simulink subsystem "IMU"  (R2025b)
settings: Solver=VariableStepAuto  StartTime=0.0  StopTime=10.0  RelTol=1e-3
libraries: simulink x1
settings Model: Creator=diego  LastModifiedBy=diego

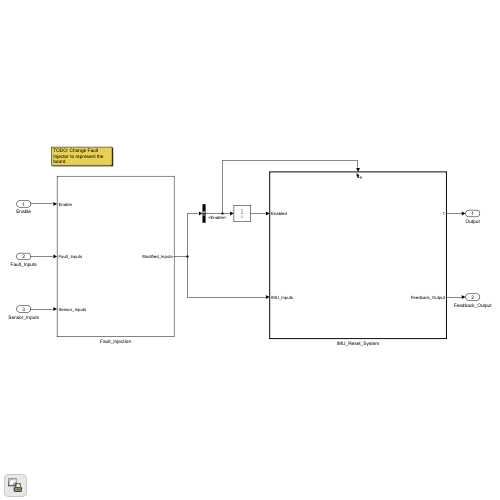
[thumbnail: Simulink's stored preview of the top-level diagram]
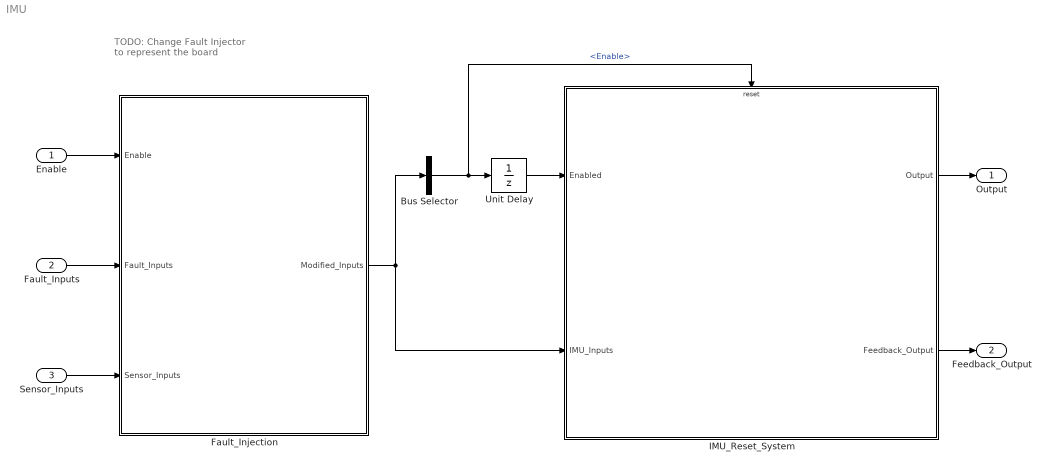
== system IMU ==
  note: TODO: Change Fault Injector to represent the board
  Enable : Inport
  Fault_Inputs : Inport  Port=2
  Sensor_Inputs : Inport  Port=3
  Bus Selector : BusSelector  OutputSignals=Enable
  Fault_Injection : Subsystem
  "IMU_Reset_System " : Subsystem  TreatAsAtomicUnit=on
  Unit Delay : UnitDelay  SampleTime=-1  HasFrameUpgradeWarning=on
  Output : Outport
  Feedback_Output : Outport  Port=2
  wires:
  Bus Selector/1 -> Unit Delay/1, "IMU_Reset_System "/Reset  "<Enable>"
  "IMU_Reset_System "/1(Output) -> Output/1
  Fault_Inputs/1 -> Fault_Injection/2(Fault_Inputs)
  Enable/1 -> Fault_Injection/1(Enable)
  Fault_Injection/1(Modified_Inputs) -> "IMU_Reset_System "/2(IMU_Inputs), Bus Selector/1
  Sensor_Inputs/1 -> Fault_Injection/3(Sensor_Inputs)
  Unit Delay/1 -> "IMU_Reset_System "/1(Enabled)
  "IMU_Reset_System "/2(Feedback_Output) -> Feedback_Output/1

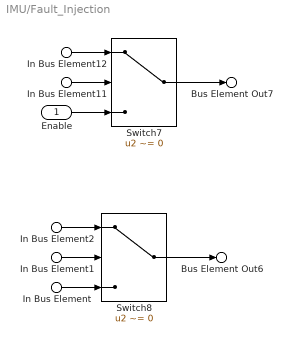
== system IMU/Fault_Injection ==
  Enable : Inport
  In Bus Element12 : Inport  Port=2  PortName=Fault_Inputs  Element=Acc_EN
  In Bus Element11 : Inport  Port=2  PortName=Fault_Inputs  Element=Override_Acc_EN
  In Bus Element1 : Inport  Port=2  PortName=Fault_Inputs  Element=Override_Wheel_Speed
  In Bus Element2 : Inport  Port=2  PortName=Fault_Inputs  Element=Wheel_Speed
  In Bus Element : Inport  Port=3  PortName=Sensor_Inputs  Element=WSS_Wheel_Speed
  Switch7 : Switch  Criteria=u2 ~= 0  SaturateOnIntegerOverflow=off  InputSameDT=off
  Switch8 : Switch  Criteria=u2 ~= 0  SaturateOnIntegerOverflow=off  InputSameDT=off
  Bus Element Out7 : Outport  PortName=Modified_Inputs  Element=Enable
  Bus Element Out6 : Outport  PortName=Modified_Inputs  Element=Wheel_Speed
  wires:
  In Bus Element2/1 -> Switch8/1
  Switch8/1 -> Bus Element Out6/1
  In Bus Element/1 -> Switch8/3
  In Bus Element1/1 -> Switch8/2
  In Bus Element12/1 -> Switch7/1
  Switch7/1 -> Bus Element Out7/1
  In Bus Element11/1 -> Switch7/2
  Enable/1 -> Switch7/3

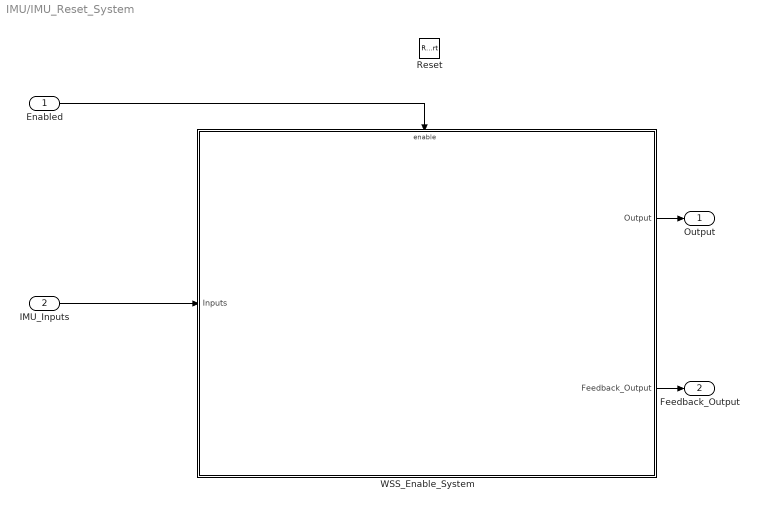
== system IMU/IMU_Reset_System  ==
  Enabled : Inport
  IMU_Inputs : Inport  Port=2
  Reset : ResetPort  DisableCoverage=on  ResetTriggerType=falling
  "WSS_Enable_System " : Subsystem  TreatAsAtomicUnit=on
  Output : Outport
  Feedback_Output : Outport  Port=2
  wires:
  "WSS_Enable_System "/2(Feedback_Output) -> Feedback_Output/1
  "WSS_Enable_System "/1(Output) -> Output/1
  IMU_Inputs/1 -> "WSS_Enable_System "/1(Inputs)
  Enabled/1 -> "WSS_Enable_System "/Enable

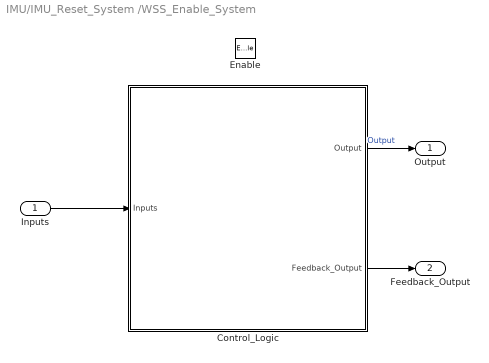
== system IMU/IMU_Reset_System /WSS_Enable_System  ==
  Inputs : Inport
  Enable : EnablePort  StatesWhenEnabling=reset
  Control_Logic : Subsystem
  Output : Outport
  Feedback_Output : Outport  Port=2
  wires:
  Control_Logic/2(Feedback_Output) -> Feedback_Output/1
  Control_Logic/1(Output) -> Output/1  "Output"
  Inputs/1 -> Control_Logic/1(Inputs)

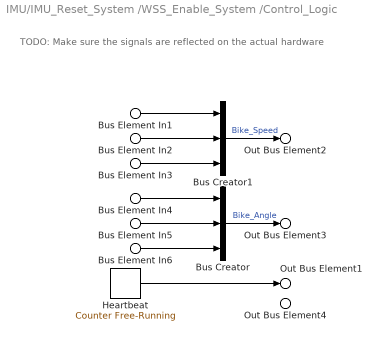
== system IMU/IMU_Reset_System /WSS_Enable_System /Control_Logic ==
  note: TODO: Make sure the signals are reflected on the actual hardware
  Bus Element In1 : Inport  PortName=Inputs  Element=Vel_X
  Bus Element In2 : Inport  PortName=Inputs  Element=Vel_Y
  Bus Element In3 : Inport  PortName=Inputs  Element=Vel_Z
  Bus Element In4 : Inport  PortName=Inputs  Element=Yaw
  Bus Element In5 : Inport  PortName=Inputs  Element=Pitch
  Bus Element In6 : Inport  PortName=Inputs  Element=Roll
  Bus Creator : BusCreator  Inputs=3
  Bus Creator1 : BusCreator  Inputs=3
  Heartbeat : simulink/Sources/Counter Free-Running  NumBits=32  tsamp=-1
  Out Bus Element1 : Outport  PortName=Output  Element=IMU_Heartbeat
  Out Bus Element2 : Outport  PortName=Output  Element=Bike_Speed
  Out Bus Element3 : Outport  PortName=Output  Element=Bike_Angle
  Out Bus Element4 : Outport  Port=2  PortName=Feedback_Output  Element=IMU_Heartbeat
  wires:
  Bus Creator/1 -> Out Bus Element3/1  "Bike_Angle"
  Bus Creator1/1 -> Out Bus Element2/1  "Bike_Speed"
  Bus Element In6/1 -> Bus Creator/3
  Bus Element In5/1 -> Bus Creator/2
  Bus Element In2/1 -> Bus Creator1/2
  Bus Element In3/1 -> Bus Creator1/3
  Bus Element In4/1 -> Bus Creator/1
  Bus Element In1/1 -> Bus Creator1/1
  Heartbeat/1 -> Out Bus Element1/1
